simulink model "Sim3"  (Simulink 7.7)
settings: Solver=ode3  StartTime=0.0  StopTime=2  FixedStep=.0001  MaxStep=.0001  RelTol=1e-3
settings Model: Creator=students  LastModifiedBy=students
settings SolverCC: MaxConsecutiveMinStep=1000

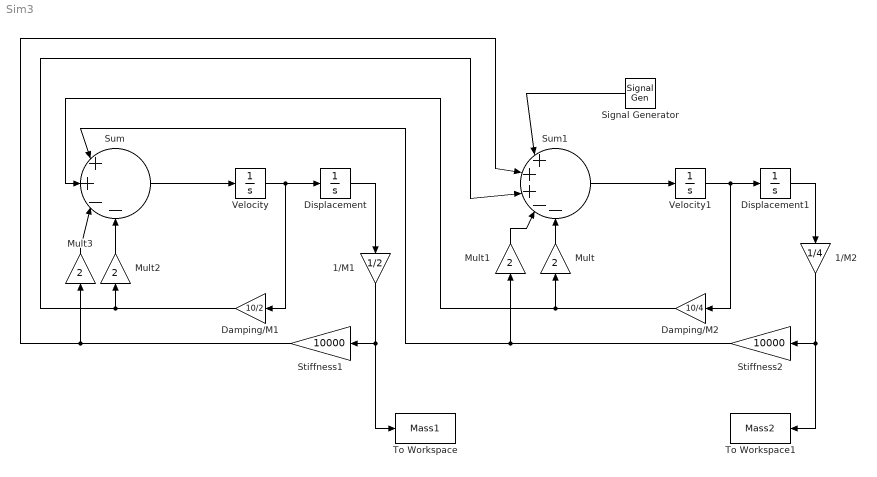
== system Sim3 ==
  1/M1 : Gain  Gain=1/2
  1/M2 : Gain  Gain=1/4
  Damping/M1 : Gain  Gain=10/2
  Damping/M2 : Gain  Gain=10/4
  Displacement : Integrator
  Displacement1 : Integrator
  Mult{,1..3} (4 alike) : Gain  Gain=2
  Signal Generator : SignalGenerator  Frequency=82.534  Units=rad/sec
  Stiffness1 : Gain  Gain=10000
  Stiffness2 : Gain  Gain=10000
  Sum : Sum  Inputs=|++--
  Sum1 : Sum  Inputs=|+++--
  To Workspace : ToWorkspace  VariableName=Mass1  SampleTime=-1  SaveFormat=Structure
  To Workspace1 : ToWorkspace  VariableName=Mass2  SampleTime=-1  SaveFormat=Structure
  Velocity : Integrator
  Velocity1 : Integrator
  wires:
  Velocity/1 -> Displacement/1, Damping/M1/1
  Displacement/1 -> 1/M1/1
  Velocity1/1 -> Damping/M2/1, Displacement1/1
  Displacement1/1 -> 1/M2/1
  Damping/M2/1 -> Sum/2, Mult/1
  Stiffness2/1 -> Sum/1, Mult1/1
  Damping/M1/1 -> Sum1/3, Mult2/1
  Stiffness1/1 -> Sum1/2, Mult3/1
  Mult/1 -> Sum1/5
  Mult2/1 -> Sum/4
  Mult3/1 -> Sum/3
  Mult1/1 -> Sum1/4
  1/M1/1 -> Stiffness1/1, To Workspace/1
  1/M2/1 -> To Workspace1/1, Stiffness2/1
  Sum/1 -> Velocity/1
  Sum1/1 -> Velocity1/1
  Signal Generator/1 -> Sum1/1
